simulink model "simulink_08_04"  (R2024a)
settings: Solver=VariableStepAuto  StartTime=0.0  StopTime=100  RelTol=1e-3
StartFcn:
  | out = [];
StopFcn:
  | try
  |     enreg = get_param('simulink_1avrilhaha/Simulateur Équipe 5', 'Enregistrement');
  |     nom = get_param('simulink_1avrilhaha/Simulateur Équipe 5', 'Fichier');
  | 
  |     if strcmp(enreg, 'on')
  |         dossier = fileparts(get_param('simulink_1avrilhaha', 'FileName'));
  | 
  |         t = out.tout;
  |         y = out.Fichier;
  | 
  |         n = min(length(t), length(y));
  |         t_cut = t(1:n);
  |         y_cut = y(1:n, :);
  | 
  |         T = table(t_cut, y_cut(:,1), 'VariableNames', {'temps', 'sortie'});
  |         writetable(T, fullfile(dossier, [nom '.csv']));
  |     end
  | catch e
  |     disp(['Erreur exportation: ' e.message]);
  | end
libraries: simulink_extras x1
settings Model: Creator=sabri  LastModifiedBy=MABRI236

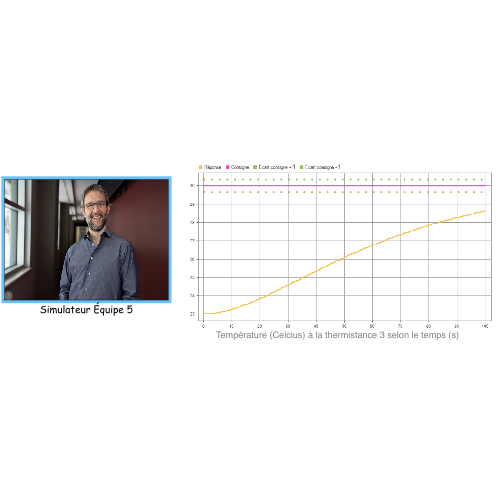
[thumbnail: Simulink's stored preview of the top-level diagram]
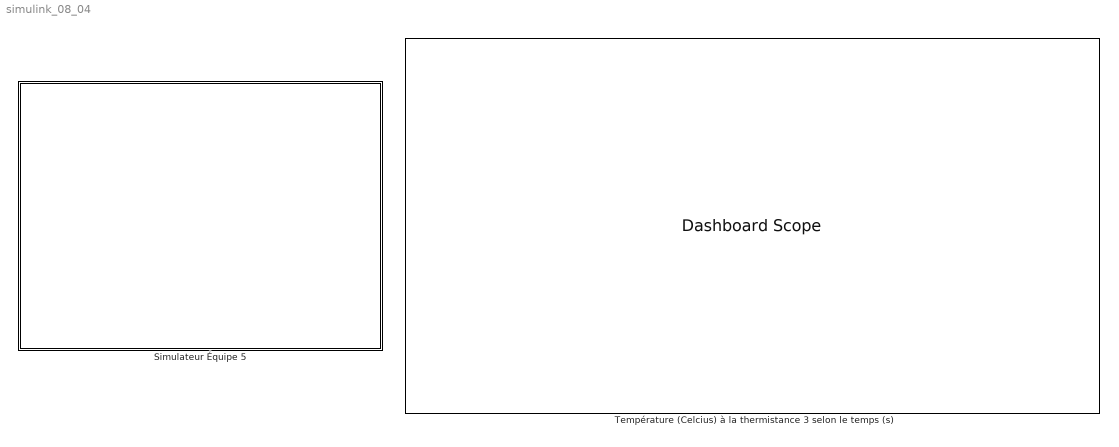
== system simulink_08_04 ==
  Simulateur Équipe 5 : Subsystem  mask{Consigne=30, T_init=23, Temps=100, Enregistrement=on, Fichier=simulation, V_2=5, V_1=1.8, R_1=3300, R_g=5600, R_f=6300, T_0=298.15, RT_0=10000, B=3900}
      mask prompts: Consigne "Température désirée"; T_init "Température initiale"; Temps "Durée de la simulation (s)"; Enregistrement "Enregistrer les données"; Fichier "Nom du fichier à enregistré:"; V_2 "Tension d'alimentation (V)"; V_1 "Tension d'alimentation de la branche positive de l'ampli-op (V)"; R_1 "Résistance de la branche négative de l'ampli-op (Ω)"; R_g "Résistance en parallèle avec la thermitance (Ω)"; R_f "Résistance du trimpot (Ω)"; T_0 "Température de référence de la thermistance (K)"; RT_0 "Résistance de référence de la thermistance (Ω)"; B "Valeur beta de la thermistance"
      mask DialogControl ParameterGroupVar Prompt: Simulateur
      mask DialogControl Container3 Prompt: Guide d'utilisation
      mask DialogControl Control2 Prompt: Voici le simulateur thermique de l'équipe 5. Vous pouvez modifier les valeurs des différents paramètres du prototype ci-dessus et choisir la température désirée.
      mask DialogControl Control3 Prompt: Lancer la simulation!
      mask DialogControl Container4 Prompt: Paramètres du prototype
      mask Display: image('4e9b43_37b74c7254004fa5961c1584dfcae1f1~mv2.jpg');
  Température (Celcius) à la thermistance 3 selon le temps (s) : DashboardScope

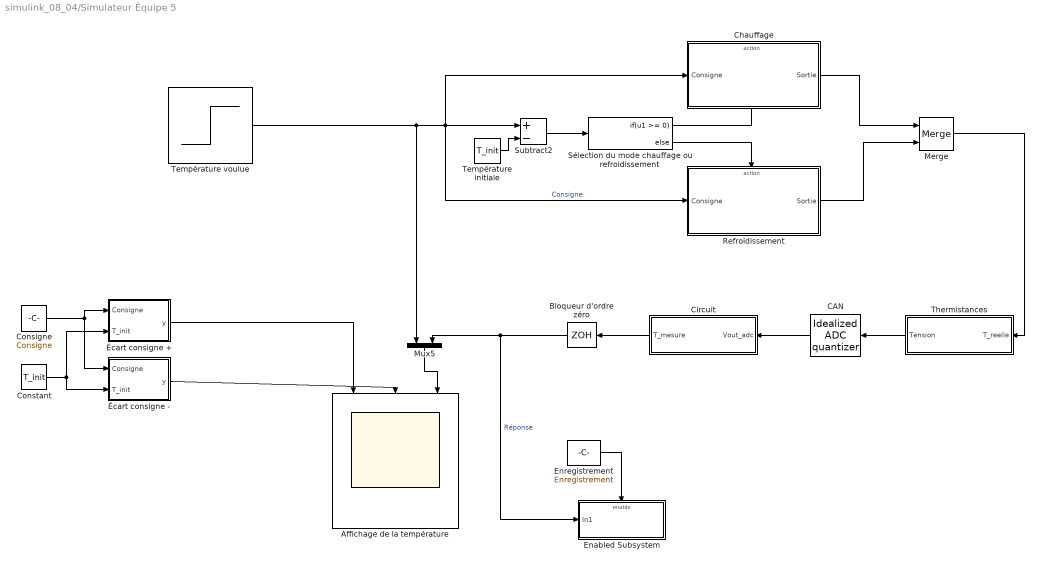
== system simulink_08_04/Simulateur Équipe 5 ==
  Affichage de la température : Scope  NumInputPorts=3
  Bloqueur d'ordre zéro : ZeroOrderHold  SampleTime=0.5
  CAN : simulink_extras/Additional Discrete/Idealized ADC quantizer  NumberOfConverterBits=10  Vmin=0  Vmax=5  OutputDataType=double  OutputNegativeValues=off
  Chauffage : Subsystem  TreatAsAtomicUnit=on
  Circuit : Subsystem
  Consigne : Constant  Value=Consigne
  Constant : Constant  Value=T_init
  Enabled Subsystem : Subsystem  TreatAsAtomicUnit=on
  Enregistrement : Constant  Value=Enregistrement
  Merge : Merge
  Mux5 : Mux  Inputs=2
  Refroidissement : Subsystem  TreatAsAtomicUnit=on
  Subtract2 : Sum  Inputs=+-
  Sélection du mode chauffage ou refroidissement : If  IfExpression=u1 >= 0
  Température initiale : Constant  Value=T_init
  Température voulue : Step  Time=0  Before=Consigne  After=Consigne  SampleTime=0
  Thermistances : Subsystem
  Écart consigne + : MATLAB Function  TreatAsAtomicUnit=on
  Écart consigne - : MATLAB Function  TreatAsAtomicUnit=on
  wires:
  Écart consigne -/1(y) -> Affichage de la température/2
  Subtract2/1 -> Sélection du mode chauffage ou refroidissement/1
  Température voulue/1 -> Refroidissement/1(Consigne), Subtract2/1, Chauffage/1(Consigne), Mux5/1  "Consigne"
  Écart consigne +/1(y) -> Affichage de la température/1
  Refroidissement/1(Sortie) -> Merge/2
  Sélection du mode chauffage ou refroidissement/1 -> Chauffage/Action
  Température initiale/1 -> Subtract2/2
  Bloqueur d'ordre zéro/1 -> Mux5/2, Enabled Subsystem/1(In1)  "Réponse"
  Thermistances/1(Tension) -> CAN/1
  Chauffage/1(Sortie) -> Merge/1
  Enregistrement/1 -> Enabled Subsystem/Enable
  Consigne/1 -> Écart consigne -/1(Consigne), Écart consigne +/1(Consigne)
  Constant/1 -> Écart consigne -/2(T_init), Écart consigne +/2(T_init)
  Mux5/1 -> Affichage de la température/3
  Merge/1 -> Thermistances/1(T_reelle)
  CAN/1 -> Circuit/1(Vout_adc)
  Circuit/1(T_mesure) -> Bloqueur d'ordre zéro/1
  Sélection du mode chauffage ou refroidissement/2 -> Refroidissement/Action

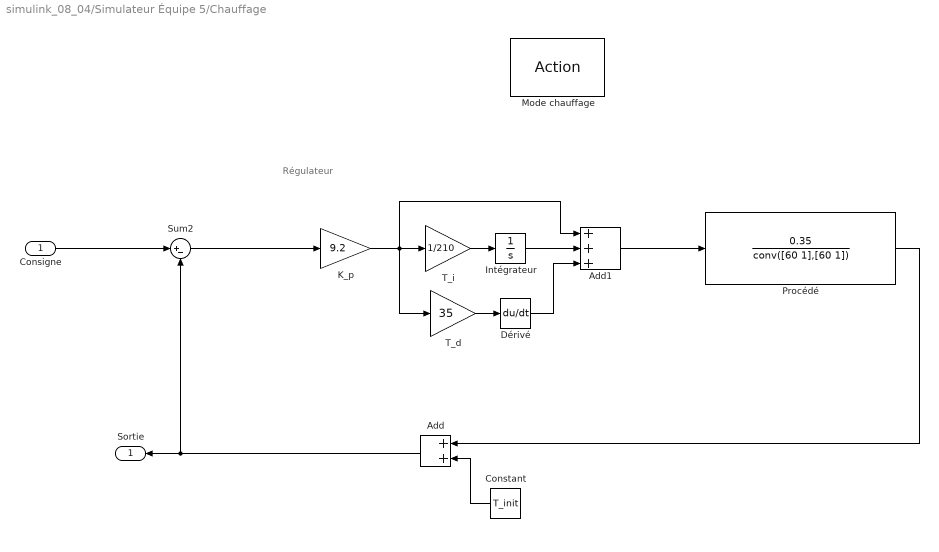
== system simulink_08_04/Simulateur Équipe 5/Chauffage ==
  note: Régulateur
  Consigne : Inport
  Mode chauffage : ActionPort  ActionPortLabel=if(u1 >= 0)
  Add : Sum
  Add1 : Sum  Inputs=+++
  Constant : Constant  Value=T_init
  Dérivé : Derivative
  Intégrateur : Integrator
  K_p : Gain  Gain=9.2
  Procédé : TransferFcn  Numerator=[0.35]  Denominator=conv([60 1],[60 1])
  Sum2 : Sum  Inputs=|+-
  T_d : Gain  Gain=35
  T_i : Gain  Gain=1/210
  Sortie : Outport
  wires:
  Sum2/1 -> K_p/1
  Intégrateur/1 -> Add1/2
  Add1/1 -> Procédé/1
  T_i/1 -> Intégrateur/1
  T_d/1 -> Dérivé/1
  Dérivé/1 -> Add1/3
  K_p/1 -> Add1/1, T_d/1, T_i/1
  Consigne/1 -> Sum2/1
  Procédé/1 -> Add/1
  Add/1 -> Sum2/2, Sortie/1
  Constant/1 -> Add/2

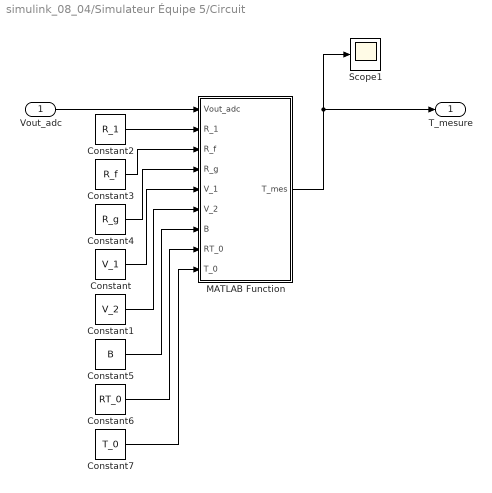
== system simulink_08_04/Simulateur Équipe 5/Circuit ==
  Vout_adc : Inport
  Constant : Constant  Value=V_1
  Constant1 : Constant  Value=V_2
  Constant2 : Constant  Value=R_1
  Constant3 : Constant  Value=R_f
  Constant4 : Constant  Value=R_g
  Constant5 : Constant  Value=B
  Constant6 : Constant  Value=RT_0
  Constant7 : Constant  Value=T_0
  MATLAB Function : MATLAB Function  TreatAsAtomicUnit=on
  Scope1 : Scope
  T_mesure : Outport
  wires:
  Vout_adc/1 -> MATLAB Function/1(Vout_adc)
  MATLAB Function/1(T_mes) -> Scope1/1, T_mesure/1
  Constant3/1 -> MATLAB Function/3(R_f)
  Constant4/1 -> MATLAB Function/4(R_g)
  Constant7/1 -> MATLAB Function/9(T_0)
  Constant/1 -> MATLAB Function/5(V_1)
  Constant1/1 -> MATLAB Function/6(V_2)
  Constant5/1 -> MATLAB Function/7(B)
  Constant6/1 -> MATLAB Function/8(RT_0)
  Constant2/1 -> MATLAB Function/2(R_1)

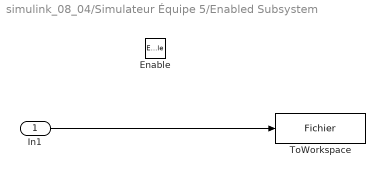
== system simulink_08_04/Simulateur Équipe 5/Enabled Subsystem ==
  In1 : Inport
  Enable : EnablePort
  ToWorkspace : ToWorkspace  VariableName=Fichier  SampleTime=0.5
  wires:
  In1/1 -> ToWorkspace/1

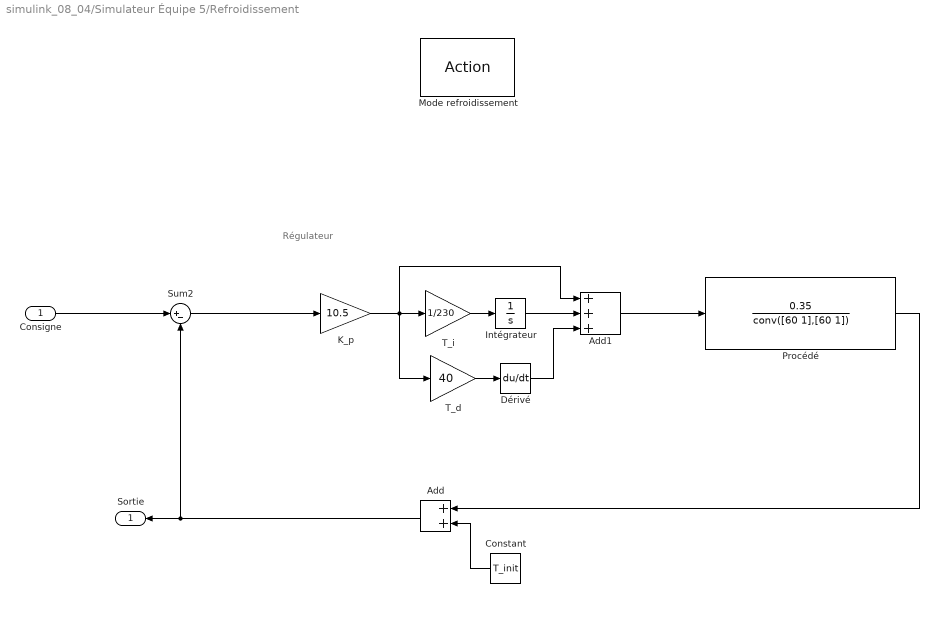
== system simulink_08_04/Simulateur Équipe 5/Refroidissement ==
  note: Régulateur
  Consigne : Inport
  Mode refroidissement : ActionPort  ActionPortLabel=else
  Add : Sum
  Add1 : Sum  Inputs=+++
  Constant : Constant  Value=T_init
  Dérivé : Derivative
  Intégrateur : Integrator
  K_p : Gain  Gain=10.5
  Procédé : TransferFcn  Numerator=[0.35]  Denominator=conv([60 1],[60 1])
  Sum2 : Sum  Inputs=|+-
  T_d : Gain  Gain=40
  T_i : Gain  Gain=1/230
  Sortie : Outport
  wires:
  Sum2/1 -> K_p/1
  K_p/1 -> Add1/1, T_d/1, T_i/1
  Procédé/1 -> Add/1
  Consigne/1 -> Sum2/1
  Intégrateur/1 -> Add1/2
  Dérivé/1 -> Add1/3
  Add/1 -> Sum2/2, Sortie/1
  T_d/1 -> Dérivé/1
  T_i/1 -> Intégrateur/1
  Add1/1 -> Procédé/1
  Constant/1 -> Add/2

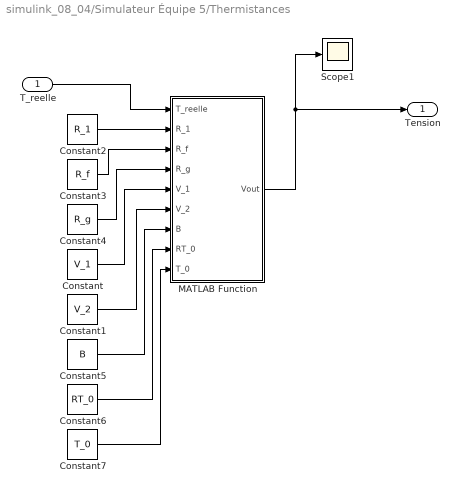
== system simulink_08_04/Simulateur Équipe 5/Thermistances ==
  T_reelle : Inport
  Constant : Constant  Value=V_1
  Constant1 : Constant  Value=V_2
  Constant2 : Constant  Value=R_1
  Constant3 : Constant  Value=R_f
  Constant4 : Constant  Value=R_g
  Constant5 : Constant  Value=B
  Constant6 : Constant  Value=RT_0
  Constant7 : Constant  Value=T_0
  MATLAB Function : MATLAB Function  TreatAsAtomicUnit=on
  Scope1 : Scope
  Tension : Outport
  wires:
  T_reelle/1 -> MATLAB Function/1(T_reelle)
  MATLAB Function/1(Vout) -> Scope1/1, Tension/1
  Constant7/1 -> MATLAB Function/9(T_0)
  Constant6/1 -> MATLAB Function/8(RT_0)
  Constant5/1 -> MATLAB Function/7(B)
  Constant1/1 -> MATLAB Function/6(V_2)
  Constant/1 -> MATLAB Function/5(V_1)
  Constant4/1 -> MATLAB Function/4(R_g)
  Constant2/1 -> MATLAB Function/2(R_1)
  Constant3/1 -> MATLAB Function/3(R_f)

== matlab function simulink_08_04/Simulateur Équipe 5/Écart consigne - ==
  data: Consigne input; y output; T_init input
function y = fcn(Consigne, T_init)

y = (-0.05*(Consigne-T_init))+Consigne;

== matlab function simulink_08_04/Simulateur Équipe 5/Écart consigne + ==
  data: Consigne input; y output; T_init input
function y = fcn(Consigne, T_init)

y = (0.05*(Consigne-T_init))+Consigne;

== matlab function simulink_08_04/Simulateur Équipe 5/Circuit/MATLAB Function ==
  data: Vout_adc input; T_mes output; R_1 input; R_f input; R_g input; V_1 input; V_2 input; B input; RT_0 input; T_0 input
function T_mes = fcn(Vout_adc, R_1, R_f, R_g, V_1, V_2, B, RT_0, T_0)
    RT = ((R_f + R_1) * R_g * V_2) / (R_1 * (5/1023)*Vout_adc + R_f * V_1) - R_g;
    T_mes = 1.0 / ((log(RT / RT_0) / B) + (1.0 / T_0)) - 273.15;
end

== matlab function simulink_08_04/Simulateur Équipe 5/Thermistances/MATLAB Function ==
  data: T_reelle input; Vout output; R_1 input; R_f input; R_g input; V_1 input; V_2 input; B input; RT_0 input; T_0 input
function Vout = fcn(T_reelle, R_1, R_f, R_g, V_1, V_2, B, RT_0, T_0)
    RT = RT_0 * exp(B * (1/(T_reelle + 273.15) - 1/T_0));
    Vout = ((R_f + R_1) * R_g * V_2) / ((RT + R_g) * R_1) - (R_f * V_1) / R_1;
end
